simulink model "Glide_3000"  (R2016b)
settings: Solver=VariableStepAuto  StartTime=0.0  StopTime=500  RelTol=1e-3
settings Model: Creator=diamond  LastModifiedBy=diamond

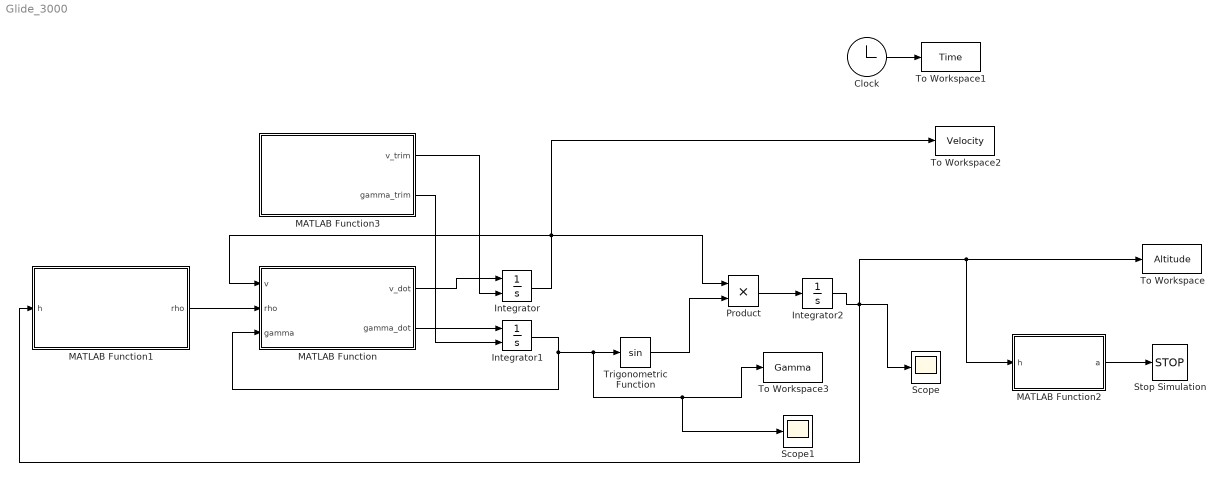
== system Glide_3000 ==
  Clock : Clock
  Integrator : Integrator  InitialConditionSource=external  InitialCondition=100
  Integrator1 : Integrator  InitialConditionSource=external  InitialCondition=-0.06
  Integrator2 : Integrator  InitialCondition=3000
  MATLAB Function : MATLAB Function  TreatAsAtomicUnit=on
  MATLAB Function1 : MATLAB Function  TreatAsAtomicUnit=on
  MATLAB Function2 : MATLAB Function  TreatAsAtomicUnit=on
  MATLAB Function3 : MATLAB Function  TreatAsAtomicUnit=on
  Product : Product
  Scope : Scope
  Scope1 : Scope
  Stop Simulation : Stop
  To Workspace : ToWorkspace  VariableName=Altitude  SaveFormat=Timeseries  SampleTime=-1
  To Workspace1 : ToWorkspace  VariableName=Time  SaveFormat=Timeseries  SampleTime=-1
  To Workspace2 : ToWorkspace  VariableName=Velocity  SaveFormat=Timeseries  SampleTime=-1
  To Workspace3 : ToWorkspace  VariableName=Gamma  SaveFormat=Timeseries  SampleTime=-1
  Trigonometric Function : Trigonometry
  wires:
  MATLAB Function/1(v_dot) -> Integrator/1
  MATLAB Function/2(gamma_dot) -> Integrator1/1
  Integrator/1 -> To Workspace2/1, Product/1, MATLAB Function/1(v)
  Integrator1/1 -> MATLAB Function/3(gamma), Scope1/1, To Workspace3/1, Trigonometric Function/1
  Trigonometric Function/1 -> Product/2
  Product/1 -> Integrator2/1
  Integrator2/1 -> Scope/1, MATLAB Function1/1(h), MATLAB Function2/1(h), To Workspace/1
  MATLAB Function1/1(rho) -> MATLAB Function/2(rho)
  Clock/1 -> To Workspace1/1
  MATLAB Function2/1(a) -> Stop Simulation/1
  MATLAB Function3/1(v_trim) -> Integrator/2
  MATLAB Function3/2(gamma_trim) -> Integrator1/2

== matlab function Glide_3000/MATLAB Function1 ==
  data: h input; rho output
function rho=func2(h)
g=9.81;
rho_sl=1.2256;
Tsl=288.15;
R=287;
T11=216.65;
rho11=0.36;
L=-0.0065;

if h<=11000
    rho=rho_sl*((Tsl + L*h)/Tsl)^(4.256);
else
    rho=rho11*exp((-g/(R*T11))*(h-11000));
end
end

== matlab function Glide_3000/MATLAB Function ==
  data: v input; v_dot output; rho input; gamma input; gamma_dot output
function [v_dot,gamma_dot]=func(v,rho,gamma)
M=70000;
g=9.81;
W=M*g;
s=122.4;
miu=0;

alpha=4*(pi/180);
Cl0=0.24;
Cl_alpha=5.19;
Cd0=0.024;
k=0.041;
Cl=Cl0+Cl_alpha*alpha;
Cd=Cd0+k*Cl^2; 
q=0.5*rho*v^2;
L=q*s*Cl;
D=q*s*Cd;
v_dot=(-D-(W*sin(gamma)))/M;
gamma_dot=(L*cos(miu)-W*cos(gamma))/(M*v);
end

== matlab function Glide_3000/MATLAB Function2 ==
  data: h input; a output
function a=func(h)
if h==0
    a=1;
else
    a=0;
end
end

== matlab function Glide_3000/MATLAB Function3 ==
  data: v_trim output; gamma_trim output
function [v_trim,gamma_trim]=func()
rho=0.9;
M=30000;
g=9.81;
W=M*g;
s=122.4;
%miu=0;

alpha=4*(pi/180);
Cl0=0.24;
Cl_alpha=5.19;
Cd0=0.024;
k=0.041;
Cl=Cl0+Cl_alpha*alpha;
Cd=Cd0+k*Cl^2; 
%q=0.5*rho*v^2;
% L=q*s*Cl;
% D=q*s*Cd;
gamma_trim=atan(Cl/Cd);
v_trim=sqrt((2*W*cos(gamma_trim))/(rho*s*Cl));
end
